simulink model "Template_no_obs2019b_v2"  (R2019b)
settings: Solver=ode1  StartTime=0.0  StopTime=inf  FixedStep=0.002  RelTol=1e-3  EnableMultiTasking=on
PostLoadFcn:
  | qc_set_target_type(getConfigSet(bdroot, 'QUARC Default Target Configuration'));
values from neighbouring files (symbols this model uses):
  Ken_eta = K(:, 4)    [LQ_KF.m]    (also in LQ_KF_version1.m; LQ_KF_version2.m = Ken(:, n+1:end); LQ_Luenberger.m; LQ_prova.m = Ken(:, n+1:end))
  Ken_x = K(:, 1:3)    [LQ_KF.m]    (also in LQ_KF_version1.m; LQ_KF_version2.m = Ken(:, 1:n); LQ_Luenberger.m; LQ_prova.m = Ken(:, 1:n))
undefined symbols (not defined in the file or in its folder): HIL, Kb, offset_corrente_volt, offset_posizione_volt, x1_eq0, x2_eq0
libraries: quarc_library x4, simulink x1
settings Model: SimulationMode=external  ExtModeTrigDuration=5000  Creator=CFulford  LastModifiedBy=Pronto all'uso
settings SolverCC: PositivePriorityOrder=on
settings DataIOCC: LimitDataPoints=on  SaveFormat=Array  SignalLoggingSaveFormat=ModelDataLogs  ReturnWorkspaceOutputs=off
settings OptimizationCC: ExpressionDepthLimit=2147483647  InitFltsAndDblsToZero=on  LifeSpan=inf
settings DebuggingCC: SaveWithParameterizedLinksMsg=none  UnderspecifiedInitializationDetection=Classic  MergeDetectMultiDrivingBlocksExec=none  SolverPrmCheckMsg=warning  MultiTaskDSMMsg=warning  MultiTaskCondExecSysMsg=none  FcnCallInpInsideContextMsg=warning  StateNameClashWarn=warning  SFUnexpectedBacktrackingDiag=warning  SFNoUnconditionalDefaultTransitionDiag=warning  SFExecutionAtInitializationDiag=none  ArithmeticOperatorsInVariantConditions=warning
settings HardwareCC: ProdBitPerPointer=32  ProdBitPerSizeT=32  ProdBitPerPtrDiffT=32  ProdLargestAtomicFloat=None  ProdIntDivRoundTo=Undefined  ProdEndianess=Unspecified  ProdWordSize=32  ProdHWDeviceType=32-bit Generic
settings ModelReferenceCC: PropagateSignalLabelsOutOfModel=off
settings SFSimCC: SimUseLocalCustomCode=off  CustomCodeUndefinedFunction=UseInterfaceOnly
settings RTWCC: Description=QUARC Win64 Target  SystemTargetFile=quarc_win64.tlc  TemplateMakefile=quarc_default_tmf  RTWUseLocalCustomCode=off
settings CodeAppCC: StateflowObjectComments=on
settings STFCustomTargetCC: TargetPreCompLibLocation=C:\PROGRA~3\QUARC\lib\2019b\win64\release  ConcurrentExecutionCompliant=on  CombineOutputUpdateFcns=on  CPPClassGenCompliant=on  SystemTargetFile=quarc_win64.tlc
settings GRTTargetCC: TargetPreCompLibLocation=C:\PROGRA~3\QUARC\lib\2019b\win64\release  TargetLangStandard=C89/C90 (ANSI)  ParMdlRefBuildCompliant=off  CompOptLevelCompliant=off  MatFileLogging=off  UseToolchainInfoCompliant=off  ExtMode=on  ExtModeMexFile=quarc_comm
settings ConfigComp: CovMetricSettings=dw  CovSaveCumulativeToWorkspaceVar=on  CovSaveSingleToWorkspaceVar=on  CovExternalEMLEnable=off  CovSFcnEnable=off

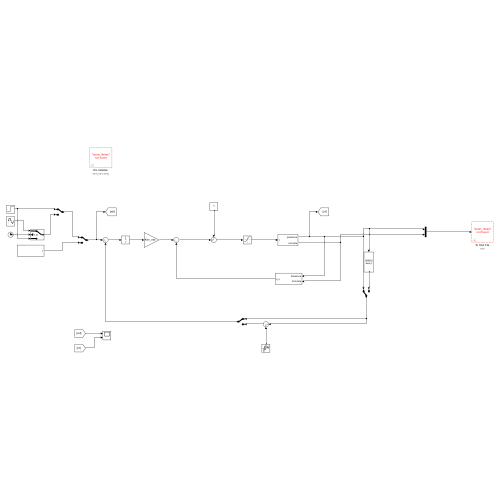
[thumbnail: Simulink's stored preview of the top-level diagram]
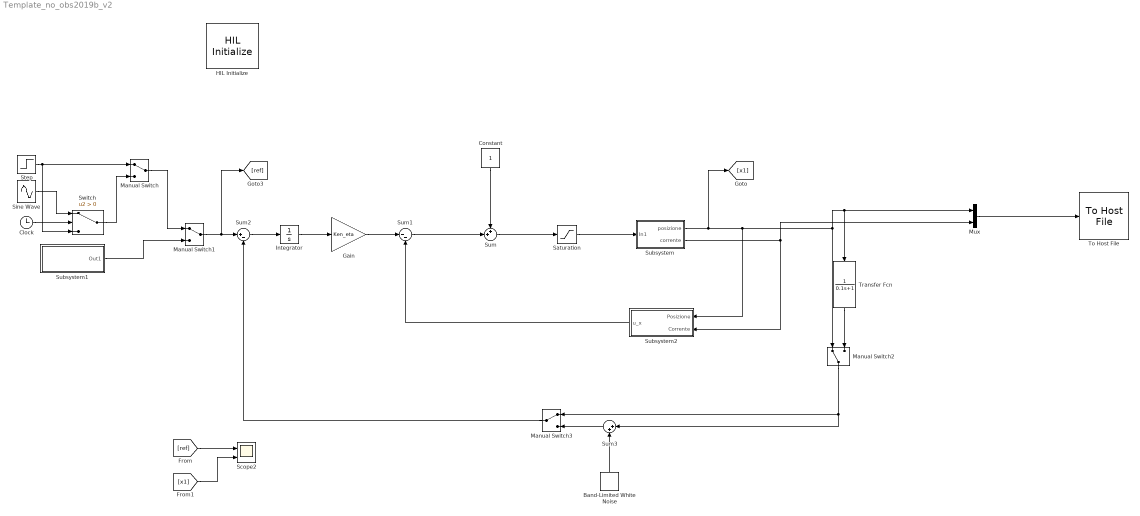
== system Template_no_obs2019b_v2 ==
  Band-Limited White Noise : simulink/Sources/Band-Limited White Noise  Cov=[8.9934e-11*0.002]  Ts=0.002  seed=[23341]
  Clock : Clock
  Constant : Constant
  Gain : Gain  Gain=Ken_eta
  HIL Initialize : quarc_library/Data Acquisition/Generic/Configuration/HIL Initialize  Priority=-99  object_name=HIL-1  board_type=q2_usb  board_number=0  board_options=d0=digital;d1=digital;led=auto;update_rate=normal;decimation=1  exclusive=off  active=off  hardware_clocks=[0]  clock_modes=[]  initial_clock_frequencies=[]  set_clock_params_at_start=off  set_clock_params_at_switch_in=off  set_clock_frequencies_at_start=off  set_clock_frequencies_at_switch_in=off  analog_input_channels=[0:1]  analog_input_configurations=[]  analog_input_maximums=10  analog_input_minimums=-10  set_analog_input_params_at_start=on  set_analog_input_params_at_switch_in=off  analog_output_channels=[0:1]  analog_output_maximums=10  analog_output_minimums=-10  initial_analog_outputs=[0]  final_analog_outputs=[0]  watchdog_analog_outputs=0  set_analog_output_params_at_start=on  set_analog_output_params_at_switch_in=off  set_analog_outputs_at_start=on  set_analog_outputs_at_switch_in=off  set_analog_outputs_at_terminate=on  set_analog_outputs_at_switch_out=off  set_analog_outputs_on_watchdog=off  digital_input_channels=[]  digital_output_channels=[]  digital_output_configuration=[]  initial_digital_outputs=[1]  final_digital_outputs=[1]  watchdog_digital_outputs=[1]  set_digital_output_params_at_start=off  set_digital_output_params_at_switch_in=off  set_digital_outputs_at_start=on  set_digital_outputs_at_switch_in=off  set_digital_outputs_at_terminate=on  set_digital_outputs_at_switch_out=off  set_digital_outputs_on_watchdog=off  encoder_channels=[0:1]  quadrature=[4]  encoder_filter_frequency=[]  initial_encoder_counts=[0]  set_encoder_params_at_start=on  set_encoder_params_at_switch_in=off  set_encoder_counts_at_start=on  set_encoder_counts_at_switch_in=off  pwm_channels=[]  pwm_modes=[0]  pwm_frequency=1/0.020  pwm_configuration=[]  pwm_alignment=[]  pwm_polarity=[]  pwm_leading_deadband=[]  pwm_trailing_deadband=[]  initial_pwm_outputs=[0]  final_pwm_outputs=[0]  watchdog_pwm_outputs=[0]  set_pwm_params_at_start=on  set_pwm_params_at_switch_in=off  set_pwm_outputs_at_start=on  set_pwm_outputs_at_switch_in=off  set_pwm_outputs_at_terminate=on  set_pwm_outputs_at_switch_out=off  set_pwm_outputs_on_watchdog=off  other_output_channels=[]  initial_other_outputs=[]  final_other_outputs=[]  watchdog_other_outputs=[]  set_other_outputs_at_start=off  set_other_outputs_at_switch_in=off  set_other_outputs_at_terminate=off  set_other_outputs_at_switch_out=off  set_other_outputs_on_watchdog=off
  Integrator : Integrator
  Manual Switch{,1..3} (4 alike) : ManualSwitch
  Mux : Mux  Inputs=2
  Saturation : Saturate  UpperLimit=23  LowerLimit=0
  Scope2 : Scope  NumInputPorts=2
  Sine Wave : Sin  Amplitude=5e-4  Bias=0.003  SampleTime=0.002
  Step : Step  Time=3  After=0.003  SampleTime=0.002
  Subsystem : Subsystem
  Subsystem1 : Subsystem
  Subsystem2 : Subsystem
  Sum : Sum  Inputs=++|
  Sum1 : Sum  Inputs=|--
  Sum2 : Sum  Inputs=|+-
  Sum3 : Sum  Inputs=|++
  Switch : Switch  Criteria=u2 > Threshold
  To Host File : quarc_library/Sinks/To Host/To Host File  file_name=data_%{date}_%{time}.mat  variable_name=data_%{date}_%{time}  decimation=1  sample_time=-1  file_format=MAT-file v.5  options=No header or footer  append=off  final_file_name=data_03-Feb-2021_14-03-21.mat  bitrate=2000000
  Transfer Fcn : TransferFcn  Denominator=[0.1 1]
  wires:
  Saturation/1 -> Subsystem/1(In1)
  Sum/1 -> Saturation/1
  Constant/1 -> Sum/1
  Sum1/1 -> Sum/2
  Gain/1 -> Sum1/1
  Integrator/1 -> Gain/1
  Sum2/1 -> Integrator/1
  Step/1 -> Switch/3, Manual Switch/1
  Sine Wave/1 -> Switch/1
  Manual Switch/1 -> Manual Switch1/1
  Subsystem1/1(Out1) -> Manual Switch1/2
  Manual Switch1/1 -> [ref], Sum2/1
  Switch/1 -> Manual Switch/2
  Clock/1 -> Switch/2
  Subsystem/2(corrente) -> Subsystem2/2(Corrente), Mux/2
  Mux/1 -> To Host File/1
  Transfer Fcn/1 -> Manual Switch2/2
  Manual Switch2/1 -> Sum3/1, Manual Switch3/1
  Subsystem2/1(u_x) -> Sum1/2
  Sum3/1 -> Manual Switch3/2
  Band-Limited White Noise/1 -> Sum3/2
  Manual Switch3/1 -> Sum2/2
  [ref] -> Scope2/1
  [x1] -> Scope2/2
  Subsystem/1(posizione) -> [x1], Subsystem2/1(Posizione), Transfer Fcn/1, Mux/1, Manual Switch2/1

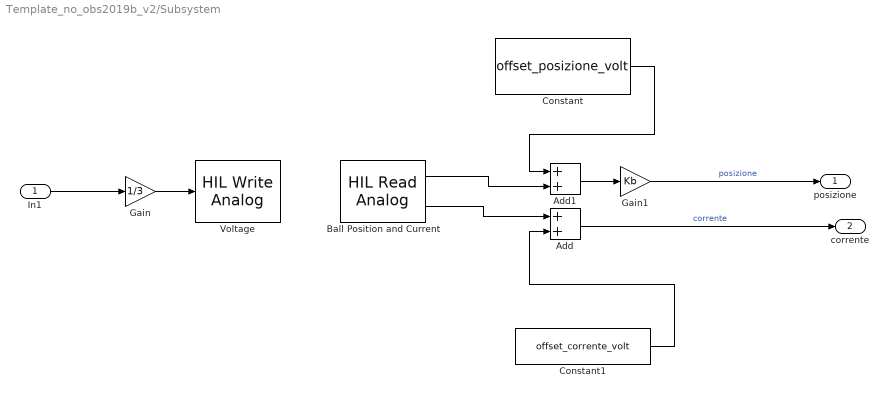
== system Template_no_obs2019b_v2/Subsystem ==
  In1 : Inport
  Add : Sum
  Add1 : Sum
  Ball Position and Current : quarc_library/Data Acquisition/Generic/Immediate I//O/HIL Read Analog  object_name=HIL-1  channels=[0:1]  sample_time=qc_get_step_size  active=on  vector_output=off
  Constant : Constant  Value=offset_posizione_volt
  Constant1 : Constant  Value=offset_corrente_volt
  Gain : Gain  Gain=1/3
  Gain1 : Gain  Gain=Kb
  Voltage : quarc_library/Data Acquisition/Generic/Immediate I//O/HIL Write Analog  object_name=HIL-1  channels=0  sample_time=-1  active=off  vector_input=off
  posizione : Outport
  corrente : Outport  Port=2
  wires:
  Add1/1 -> Gain1/1
  Constant1/1 -> Add/2
  Ball Position and Current/1 -> Add1/2
  Ball Position and Current/2 -> Add/1
  Constant/1 -> Add1/1
  Gain/1 -> Voltage/1
  In1/1 -> Gain/1
  Gain1/1 -> posizione/1  "posizione"
  Add/1 -> corrente/1  "corrente"

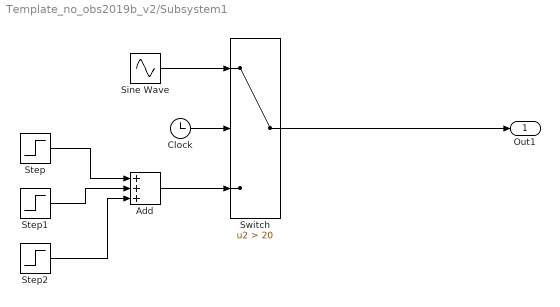
== system Template_no_obs2019b_v2/Subsystem1 ==
  Add : Sum  Inputs=+++
  Clock : Clock
  Sine Wave : Sin  Amplitude=0.002  Bias=0.005  SampleTime=0.002
  Step : Step  Time=3  After=0.003  SampleTime=0.002
  Step1 : Step  Time=5  After=0.004  SampleTime=0.002
  Step2 : Step  Time=10  After=-0.002  SampleTime=0.002
  Switch : Switch  Criteria=u2 > Threshold  Threshold=20
  Out1 : Outport
  wires:
  Switch/1 -> Out1/1
  Step/1 -> Add/1
  Step1/1 -> Add/2
  Step2/1 -> Add/3
  Add/1 -> Switch/3
  Clock/1 -> Switch/2
  Sine Wave/1 -> Switch/1

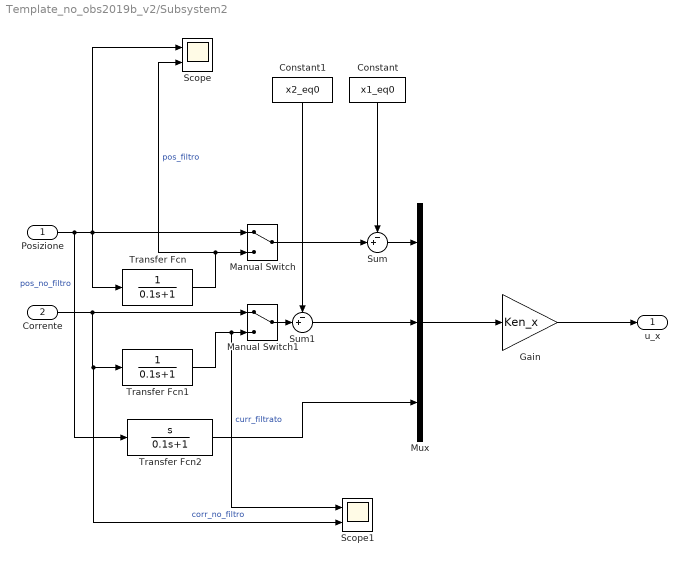
== system Template_no_obs2019b_v2/Subsystem2 ==
  Posizione : Inport
  Corrente : Inport  Port=2
  Constant : Constant  Value=x1_eq0
  Constant1 : Constant  Value=x2_eq0
  Gain : Gain  Gain=Ken_x
  Manual Switch : ManualSwitch
  Manual Switch1 : ManualSwitch
  Mux : Mux  Inputs=3
  Scope : Scope  NumInputPorts=2
  Scope1 : Scope  NumInputPorts=2
  Sum : Sum  Inputs=-+|
  Sum1 : Sum  Inputs=-+|
  Transfer Fcn : TransferFcn  Denominator=[0.1 1]
  Transfer Fcn1 : TransferFcn  Denominator=[0.1 1]
  Transfer Fcn2 : TransferFcn  Numerator=[1 0]  Denominator=[0.1 1]
  u_x : Outport
  wires:
  Posizione/1 -> Transfer Fcn2/1, Scope/1, Transfer Fcn/1, Manual Switch/1  "pos_no_filtro"
  Gain/1 -> u_x/1
  Constant/1 -> Sum/1
  Sum/1 -> Mux/1
  Transfer Fcn2/1 -> Mux/3
  Mux/1 -> Gain/1
  Manual Switch/1 -> Sum/2
  Sum1/1 -> Mux/2
  Corrente/1 -> Scope1/2, Transfer Fcn1/1, Manual Switch1/1  "corr_no_filtro"
  Manual Switch1/1 -> Sum1/2
  Constant1/1 -> Sum1/1
  Transfer Fcn1/1 -> Scope1/1, Manual Switch1/2  "curr_filtrato"
  Transfer Fcn/1 -> Manual Switch/2, Scope/2  "pos_filtro"
